simulink model "Interpolator"  (R2018b)
settings: Solver=FixedStepAuto  StartTime=0.0  StopTime=10.0  FixedStep=0.001  RelTol=1e-3
settings Model: Creator=EiLit  LastModifiedBy=EiLit

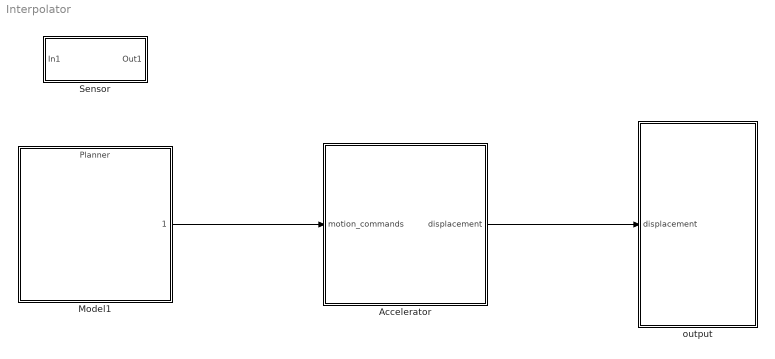
== system Interpolator ==
  Accelerator : Subsystem
  Model1 : ModelReference  ModelNameDialog=Planner  SimulationMode=Normal  ModelReferenceVersion=1.2
  Sensor : Subsystem
  output : Subsystem
  wires:
  Model1/1 -> Accelerator/1(motion_commands)
  Accelerator/1(displacement) -> output/1(displacement)

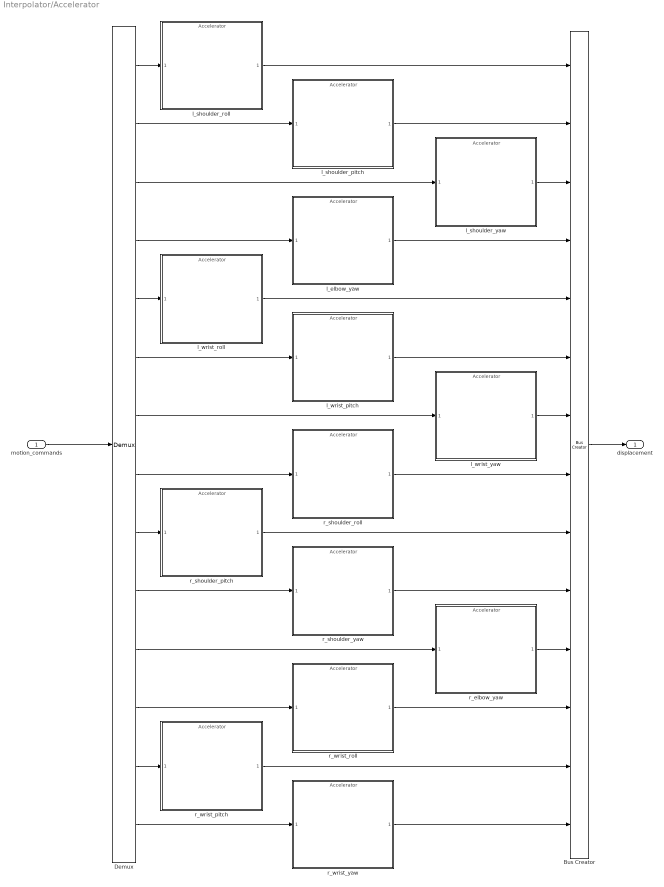
== system Interpolator/Accelerator ==
  motion_commands : Inport
  Bus Creator : BusCreator  Inputs=14
  Demux : Demux  Outputs=14
  l_elbow_yaw : ModelReference  ModelNameDialog=Accelerator  SimulationMode=Normal  ModelReferenceVersion=1.21
  l_shoulder_pitch : ModelReference  ModelNameDialog=Accelerator  SimulationMode=Normal  ModelReferenceVersion=1.21
  l_shoulder_roll : ModelReference  ModelNameDialog=Accelerator  SimulationMode=Normal  ModelReferenceVersion=1.21
  l_shoulder_yaw : ModelReference  ModelNameDialog=Accelerator  SimulationMode=Normal  ModelReferenceVersion=1.21
  l_wrist_pitch : ModelReference  ModelNameDialog=Accelerator  SimulationMode=Normal  ModelReferenceVersion=1.21
  l_wrist_roll : ModelReference  ModelNameDialog=Accelerator  SimulationMode=Normal  ModelReferenceVersion=1.21
  l_wrist_yaw : ModelReference  ModelNameDialog=Accelerator  SimulationMode=Normal  ModelReferenceVersion=1.21
  r_elbow_yaw : ModelReference  ModelNameDialog=Accelerator  SimulationMode=Normal  ModelReferenceVersion=1.21
  r_shoulder_pitch : ModelReference  ModelNameDialog=Accelerator  SimulationMode=Normal  ModelReferenceVersion=1.21
  r_shoulder_roll : ModelReference  ModelNameDialog=Accelerator  SimulationMode=Normal  ModelReferenceVersion=1.21
  r_shoulder_yaw : ModelReference  ModelNameDialog=Accelerator  SimulationMode=Normal  ModelReferenceVersion=1.21
  r_wrist_pitch : ModelReference  ModelNameDialog=Accelerator  SimulationMode=Normal  ModelReferenceVersion=1.21
  r_wrist_roll : ModelReference  ModelNameDialog=Accelerator  SimulationMode=Normal  ModelReferenceVersion=1.21
  r_wrist_yaw : ModelReference  ModelNameDialog=Accelerator  SimulationMode=Normal  ModelReferenceVersion=1.21
  displacement : Outport
  wires:
  motion_commands/1 -> Demux/1
  Demux/1 -> l_shoulder_roll/1
  Demux/2 -> l_shoulder_pitch/1
  Demux/3 -> l_shoulder_yaw/1
  Demux/4 -> l_elbow_yaw/1
  Demux/5 -> l_wrist_roll/1
  Demux/7 -> l_wrist_yaw/1
  Demux/6 -> l_wrist_pitch/1
  Demux/8 -> r_shoulder_roll/1
  Demux/9 -> r_shoulder_pitch/1
  Demux/10 -> r_shoulder_yaw/1
  Demux/11 -> r_elbow_yaw/1
  Demux/12 -> r_wrist_roll/1
  Demux/13 -> r_wrist_pitch/1
  Demux/14 -> r_wrist_yaw/1
  r_wrist_yaw/1 -> Bus Creator/14
  r_wrist_pitch/1 -> Bus Creator/13
  r_wrist_roll/1 -> Bus Creator/12
  r_elbow_yaw/1 -> Bus Creator/11
  r_shoulder_yaw/1 -> Bus Creator/10
  r_shoulder_pitch/1 -> Bus Creator/9
  r_shoulder_roll/1 -> Bus Creator/8
  l_wrist_yaw/1 -> Bus Creator/7
  l_wrist_pitch/1 -> Bus Creator/6
  l_wrist_roll/1 -> Bus Creator/5
  l_elbow_yaw/1 -> Bus Creator/4
  l_shoulder_yaw/1 -> Bus Creator/3
  l_shoulder_pitch/1 -> Bus Creator/2
  l_shoulder_roll/1 -> Bus Creator/1
  Bus Creator/1 -> displacement/1

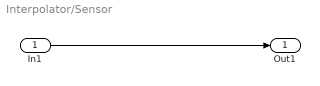
== system Interpolator/Sensor ==
  In1 : Inport
  Out1 : Outport
  wires:
  In1/1 -> Out1/1

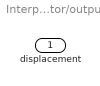
== system Interpolator/output ==
  displacement : Inport
